simulink model "virtual_wheel_damping_discrete"  (R2020a)
settings: Solver=ode4  StartTime=0.0  StopTime=tfinal  FixedStep=Deltat  RelTol=1e-3  EnableMultiTasking=on
values from neighbouring files (symbols this model uses):
  b = ????    [virtual_wheel_noJbk.m]
  Jw = ????    [virtual_wheel_noJbk.m]
  k = ?????    [virtual_wheel_noJbk.m]
  step_time = 1    [virtual_wheel_noJbk.m]
  T = .001    (= 0.001)    [virtual_wheel_noJbk.m]
  Theta_z_0 = 45    [virtual_wheel_noJbk.m]
undefined symbols (not defined in the file or in its folder): DiscIntNeverNeededParam
settings Model: ExtModeTrigMode=oneshot  ExtModeArmWhenConnect=off  Creator=jfr  LastModifiedBy=jfr
settings DataIOCC: SaveFormat=Array  SignalLoggingSaveFormat=ModelDataLogs  ReturnWorkspaceOutputs=off  SignalLoggingName=sigsOut
settings OptimizationCC: BooleanDataType=off  InitFltsAndDblsToZero=on  LifeSpan=inf
settings DebuggingCC: SaveWithParameterizedLinksMsg=none  UnderspecifiedInitializationDetection=Classic  MergeDetectMultiDrivingBlocksExec=none  SignalResolutionControl=TryResolveAllWithWarning  MultiTaskDSMMsg=warning  MultiTaskCondExecSysMsg=none  AllowSymbolicDim=off  SFUnexpectedBacktrackingDiag=warning  SFNoUnconditionalDefaultTransitionDiag=warning  SFExecutionAtInitializationDiag=none  ArithmeticOperatorsInVariantConditions=warning
settings HardwareCC: ProdBitPerPointer=32  ProdBitPerSizeT=32  ProdBitPerPtrDiffT=32  ProdLargestAtomicFloat=None  ProdIntDivRoundTo=Undefined  ProdEndianess=Unspecified  ProdWordSize=32  ProdHWDeviceType=32-bit Generic  TargetUnknown=on
settings ModelReferenceCC: PropagateSignalLabelsOutOfModel=off
settings SFSimCC: SimUseLocalCustomCode=off  CustomCodeUndefinedFunction=UseInterfaceOnly
settings RTWCC: RTWUseLocalCustomCode=off
settings CodeAppCC: StateflowObjectComments=on
settings GRTTargetCC: TargetFcnLib=ansi_tfl_tmw.mat  TargetLangStandard=C89/C90 (ANSI)  ModelReferenceCompliant=off  CombineOutputUpdateFcns=off  MatFileLogging=off  GRTInterface=on
settings ConfigComp: CovMetricSettings=dw  CovHtmlReporting=on  CovSaveCumulativeToWorkspaceVar=on  CovSaveSingleToWorkspaceVar=on  CovExternalEMLEnable=off

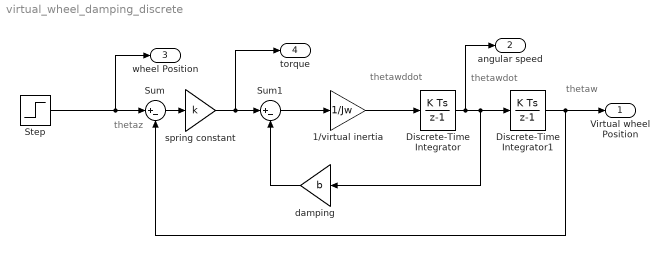
== system virtual_wheel_damping_discrete ==
  note: thetaw
  note: thetawdot
  note: thetawddot
  note: thetaz
  1/virtual inertia : Gain  Gain=1/Jw  SaturateOnIntegerOverflow=on  OutDataTypeStr=Inherit: Same as input  ParamDataTypeStr=Inherit: Same as input
  Discrete-Time Integrator : DiscreteIntegrator  SampleTime=T  ICPrevOutput=DiscIntNeverNeededParam  ICPrevScaledInput=DiscIntNeverNeededParam
  Discrete-Time Integrator1 : DiscreteIntegrator  SampleTime=T  ICPrevOutput=DiscIntNeverNeededParam  ICPrevScaledInput=DiscIntNeverNeededParam
  Step : Step  Time=step_time  After=Theta_z_0  SampleTime=0
  Sum : Sum  Inputs=|+-  InputSameDT=on  SaturateOnIntegerOverflow=on  OutDataTypeStr=Inherit: Same as first input
  Sum1 : Sum  Inputs=|+-  InputSameDT=on  SaturateOnIntegerOverflow=on  OutDataTypeStr=Inherit: Same as first input
  damping : Gain  Gain=b  SaturateOnIntegerOverflow=on  OutDataTypeStr=Inherit: Same as input  ParamDataTypeStr=Inherit: Same as input
  spring constant : Gain  Gain=k  SaturateOnIntegerOverflow=on  OutDataTypeStr=Inherit: Same as input  ParamDataTypeStr=Inherit: Same as input
  Virtual wheel Position : Outport  VectorParamsAs1DForOutWhenUnconnected=off
  angular speed : Outport  Port=2  VectorParamsAs1DForOutWhenUnconnected=off
  wheel Position : Outport  Port=3  VectorParamsAs1DForOutWhenUnconnected=off
  torque : Outport  Port=4  VectorParamsAs1DForOutWhenUnconnected=off
  wires:
  Discrete-Time Integrator1/1 -> Virtual wheel Position/1, Sum/2
  Sum/1 -> spring constant/1
  Step/1 -> wheel Position/1, Sum/1
  spring constant/1 -> torque/1, Sum1/1
  1/virtual inertia/1 -> Discrete-Time Integrator/1
  Discrete-Time Integrator/1 -> angular speed/1, damping/1, Discrete-Time Integrator1/1
  Sum1/1 -> 1/virtual inertia/1
  damping/1 -> Sum1/2
